simulink model "VTOLTiltrotor"  (R2024b)
settings: configuration reference "VTOLConfiguration" (kept outside this file)
undefined symbols (not defined in the file): airspeed, CityMission, ddx, ddy, ddz, dx, dy, dz, Earth, FixedWingMission, fractalcoef, HoverMission, p, params, pitch, position, q, r, roll, SensorAAFiltDen, SensorAAFiltNum, TransitionMission, UAVSampleTime, WGS84, X, Y, yaw, Z
libraries: robotcorelib x3, simulink x2, mspfiltlib x1, simulink_extras x1, aerolibtransform2 x1, aerolibatmos2 x1, sensorgpslib x1, mspsensorlib x1, sim3dlib x1, uavsim3dlib x1, uavutilslib x1
settings Model: DataDictionary=VTOLDynamicsData.sldd  PauseTimes=13.8  Creator=The MathWorks, Inc.  LastModifiedBy=mhcho
settings ConfigSetRef: SourceName=VTOLConfiguration

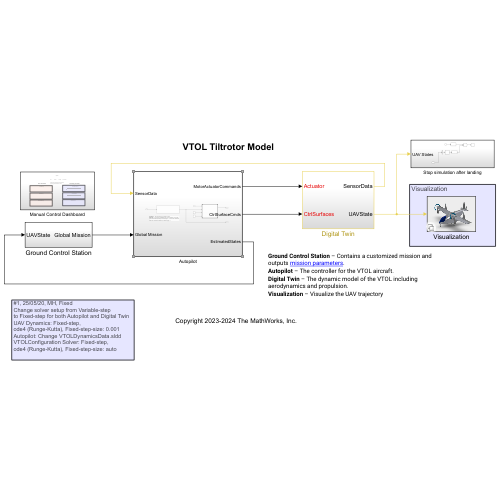
[thumbnail: Simulink's stored preview of the top-level diagram]
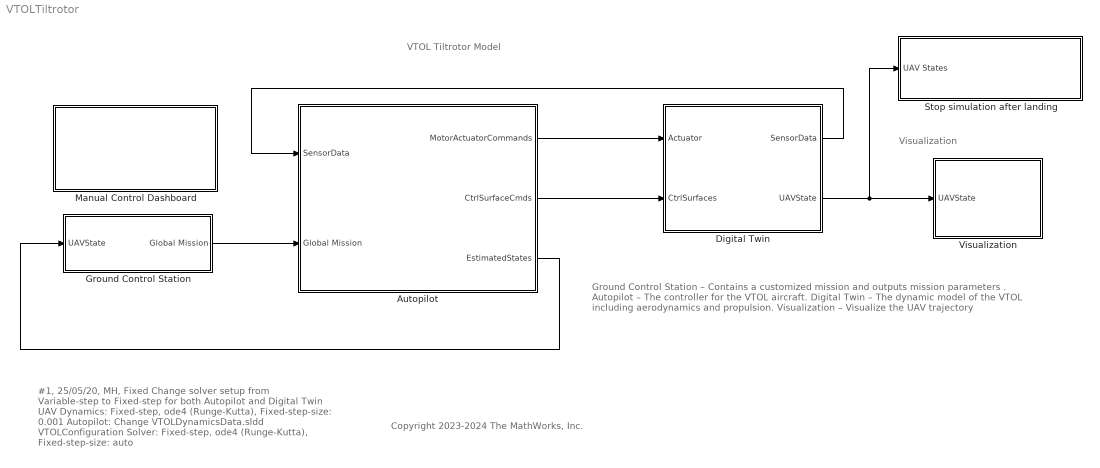
== system VTOLTiltrotor ==
  note: Ground Control Station – Contains a customized mission and outputs mission parameters .
      | Autopilot – The controller for the VTOL aircraft.
      | Digital Twin – The dynamic model of the VTOL including aerodynamics and propulsion.
      | Visualization – Visualize the UAV trajectory
  note: VTOL Tiltrotor Model
  note: Visualization
  note: Copyright 2023-2024 The MathWorks, Inc.
  note: #1, 25/05/20, MH, Fixed
      | Change solver setup from Variable-step
      | to Fixed-step for both Autopilot and Digital Twin
      | UAV Dynamics: Fixed-step,
      | ode4 (Runge-Kutta), Fixed-step-size: 0.001
      | Autopilot: Change VTOLDynamicsData.sldd
      | VTOLConfiguration Solver: Fixed-step,
      | ode4 (Runge-Kutta), Fixed-step-size: auto
  Autopilot : Subsystem
  Digital Twin : Subsystem
  Ground Control Station : Subsystem
  Manual Control Dashboard : Subsystem
  Stop simulation after landing : Subsystem
  Visualization : Subsystem  Variant=on  VariantControl=Visualization
      mask Display: image('TiltrotorVisualization.PNG'); % Use "Edit Image" on toolstrip to change.
  wires:
  Digital Twin/2(UAVState) -> Stop simulation after landing/1(UAV States), Visualization/1(UAVState)
  Ground Control Station/1(Global Mission) -> Autopilot/2(Global Mission)
  Autopilot/3(EstimatedStates) -> Ground Control Station/1(UAVState)
  Digital Twin/1(SensorData) -> Autopilot/1(SensorData)
  Autopilot/1(MotorActuatorCommands) -> Digital Twin/1(Actuator)
  Autopilot/2(CtrlSurfaceCmds) -> Digital Twin/2(CtrlSurfaces)

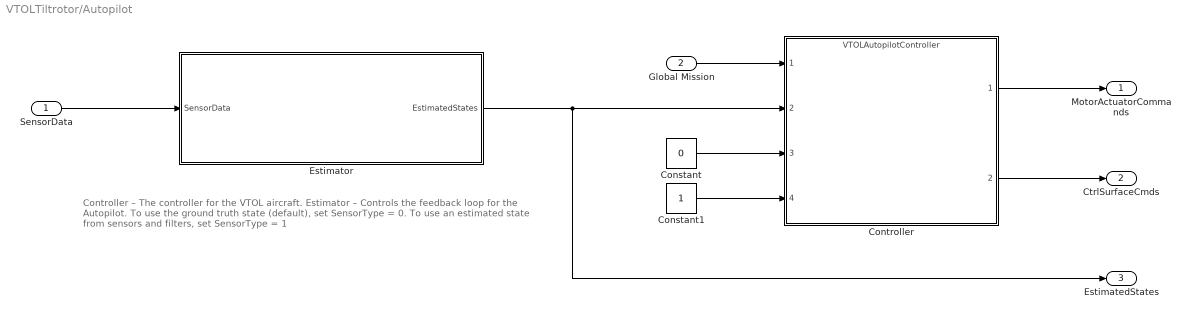
== system VTOLTiltrotor/Autopilot ==
  note: Controller – The controller for the VTOL aircraft.
      | Estimator – Controls the feedback loop for the Autopilot. To use the ground truth state (default), set SensorType = 0. To use an estimated state from sensors and filters, set SensorType = 1
  SensorData : Inport
  Global Mission : Inport  Port=2
  Constant : Constant  Value=0
  Constant1 : Constant
  Controller : ModelReference  ModelNameDialog=VTOLAutopilotController  SimulationMode=Normal  ModelReferenceVersion=1.218
  Estimator : Subsystem  Variant=on
  MotorActuatorCommands : Outport
  CtrlSurfaceCmds : Outport  Port=2
  EstimatedStates : Outport  Port=3
  wires:
  Estimator/1(EstimatedStates) -> EstimatedStates/1, Controller/2
  Controller/1 -> MotorActuatorCommands/1
  SensorData/1 -> Estimator/1(SensorData)
  Controller/2 -> CtrlSurfaceCmds/1
  Global Mission/1 -> Controller/1
  Constant/1 -> Controller/3
  Constant1/1 -> Controller/4

== system VTOLTiltrotor/Digital Twin ==
  Actuator : Inport
  CtrlSurfaces : Inport  Port=2
  Rate Transition : RateTransition
  Rate Transition1 : RateTransition
  To Workspace : ToWorkspace  VariableName=UAV_State  SaveFormat=Timeseries  SampleTime=-1
  UAV Dynamics : ModelReference  ModelNameDialog=VTOLDynamics  SimulationMode=Normal  ModelReferenceVersion=1.74
  Variant Subsystem : Subsystem  Variant=on  VariantControl=Choice
  SensorData : Outport
  UAVState : Outport  Port=2
  wires:
  Variant Subsystem/1(SensorData) -> SensorData/1
  UAV Dynamics/1 -> To Workspace/1, Variant Subsystem/1(UAVStates), UAVState/1  "Ground Truth"
  Actuator/1 -> Rate Transition/1
  CtrlSurfaces/1 -> Rate Transition1/1
  Rate Transition/1 -> UAV Dynamics/1
  Rate Transition1/1 -> UAV Dynamics/2

== system VTOLTiltrotor/Ground Control Station ==
  note: Set mission type. In the project shortcut, choose between:
      | Hover mission by selecting Guidance Mode under Hover
      | Fixed wing mission by selecting Guidance Mode under Fixed wing
      | Transition mission by selecting Set Up Full Transition Mission under Transition
      | City mission by selecting Set Up City Mission under Photorealistic Simulation
  UAVState : Inport
  Get Flight Mission : Subsystem  Variant=on  VariantControlMode=label  LabelModeActiveChoice=useQGC==0
  Global Mission : Outport  SampleTime=0.005
  wires:
  UAVState/1 -> Get Flight Mission/1(UAVState)
  Get Flight Mission/1("Mission ") -> Global Mission/1

== system VTOLTiltrotor/Manual Control Dashboard ==
  note: Commanded Altitude
  note: Flight Mode
  note: Commanded Y (m)
  note: Fixed Wing
  note: Commanded Airspeed (m)
  note: Hover
  note: Transition
  note: Commanded Course
  note: Fixed Wing Commands
  note: Hover Commands
  note: Commanded Altitude (m)
  note: Back Transition
  note: Commanded X (m)
  note: Change these parameters during simulation when using manual testbench mode.
  FlightModeSlider : SliderBlock  LabelPosition=Hide  ScaleMax=3  TickInterval=1
  Slider1 : SliderBlock  LabelPosition=Hide  ScaleMax=50  TickInterval=5
  Slider2 : SliderBlock  LabelPosition=Hide  ScaleMin=-30  ScaleMax=30  TickInterval=5
  Slider3 : SliderBlock  LabelPosition=Hide  ScaleMin=-30  ScaleMax=30  TickInterval=5
  Slider5 : SliderBlock  LabelPosition=Hide  ScaleMin=-30  ScaleMax=30  TickInterval=5
  Slider6 : SliderBlock  LabelPosition=Hide  ScaleMin=-100  TickInterval=10
  Slider7 : SliderBlock  LabelPosition=Hide  ScaleMin=10  ScaleMax=30  TickInterval=5

== system VTOLTiltrotor/Stop simulation after landing ==
  UAV States : Inport
  AND : Logic  IconShape=distinctive  AllPortsSameDT=off  OutDataTypeStr=boolean
  Bus Selector : BusSelector  OutputSignals=Xe
  Clock : Clock
  Compare To Constant : simulink/Logic and Bit Operations/Compare To Constant  relop=>=  const=-1e-2  OutDataTypeStr=boolean
  Compare To Constant1 : simulink/Logic and Bit Operations/Compare To Constant  relop=>=  const=5  OutDataTypeStr=boolean
  Selector : Selector  InputPortWidth=3  IndexOptions=Index vector (dialog)  Indices=3  OutputSizes=1
  Stop Simulation : Stop
  wires:
  Bus Selector/1 -> Selector/1  "<Xe>"
  AND/1 -> Stop Simulation/1
  Compare To Constant1/1 -> AND/1
  UAV States/1 -> Bus Selector/1
  Clock/1 -> Compare To Constant1/1
  Compare To Constant/1 -> AND/2
  Selector/1 -> Compare To Constant/1

== system VTOLTiltrotor/Visualization ==
  UAVState : Inport
  No Visualization : Subsystem  VariantControl=Visualization==0
  Photorealistic : Subsystem  VariantControl=Visualization==2
  Visualization : Subsystem  VariantControl=Visualization==1

== system VTOLTiltrotor/Autopilot/Estimator ==
  SensorData : Inport
  Estimation Filter : Subsystem  VariantControl=SensorType==1
  Ground Truth : Subsystem  VariantControl=SensorType==0
  EstimatedStates : Outport

== system VTOLTiltrotor/Digital Twin/Variant Subsystem ==
  UAVStates : Inport
  No Sensors : Subsystem  VariantControl=SensorType==0
  Sensors : Subsystem  VariantControl=SensorType==1
  SensorData : Outport

== system VTOLTiltrotor/Ground Control Station/Get Flight Mission ==
  UAVState : Inport
  noQGC : Subsystem  TreatAsAtomicUnit=on  SystemSampleTime=UAVSampleTime*4  VariantControl=useQGC==0
  "Mission " : Outport

== system VTOLTiltrotor/Visualization/No Visualization ==
  UAVState : Inport
  Terminator : Terminator
  wires:
  UAVState/1 -> Terminator/1

== system VTOLTiltrotor/Visualization/Photorealistic ==
  UAVState : Inport
  Bus Creator : BusCreator  Inputs=6
  Bus Selector : BusSelector  OutputSignals=Euler,Xe
  Demux : Demux  Outputs=3
  Demux1 : Demux  Outputs=3
  Prepare UAV Data : Subsystem
  Simulation 3D Scene Configuration : sim3dlib/Simulation 3D Scene Configuration  Priority=0  ProjectFormat=Unreal Editor  SceneDesc=US city block  ProjectName=I:\29\vdubey.MergedFixedWingReview\matlab\toolbox\shared\sim3d_projects\automotive_project_windows\UE\WindowsNoEditor\VehicleSimulation.exe  ScenePath=/Game/Maps/USCityBlock  UEProjPath=C:\project\AutoVrtlEnv\AutoVrtlEnv.uproject  EnableOpenDRIVE=off  vehTagList={'Custom';'Scene Origin';'VTOL_Vehicle'}  vehTag=VTOL_Vehicle  FreeCameraInitialTranslation=[0, 0, 0]  FreeCameraDefaultInitialTranslation=[-6, 0, 2]  FreeCameraInitialRotation=[0, 0, 0]  FreeCameraDefaultInitialRotation=[0, -15, 0]  OpVisEn=off  Ts=1/10  EnableWindow=on  EnableRemoteAccess=off  EnableWeather=off  SunAzimuth=90  SunAltitude=40.0  EnableGeospatialSun=off  Latitude=0  Longitude=0  Date=2023-01-01  Time=10:30:00  GeoTimeZone=-5.0  SunDaylightSaving=off  wind=1  clouds=10  EnableVolumetricClouds=off  CloudCoverage=0  CloudAltitude=6  fog=0  rain=0  RaindropsEffect=off  SnowDensity=0  EnableGeospatial=off  UseTrueOrigin=off  OriginHeight=200  OriginLatitude=40.744652  OriginLongitude=-73.988864  MapStyle=Aerial  AdditionalAssetIDs=[]  UseAdvancedSunSky=off  SolarTime=11  TimeZone=-5  Day=21  Month=9  Year=2022  UseDaylightSavingTime=on  DSTStartDay=10  DSTStartMonth=3  DSTEndDay=3  DSTEndMonth=11  DSTSwitchHour=2  sensorTag=MainCamera2  sensorId=2  sensorName=MainCamera2  mountLoc=Origin  offsetFlag=off  tmountOffset=[0, 0, 0]  rmountOffset=[0, 0, 0]  HorizontalResolution=1280  VerticalResolution=720  HorizontalFOV=60  mountPoint=[0 0 0]  mountOrientation=[0 0 0]  aMode=4  ID=2  GeoTrigger=Inactive
      settings: LibrarySourceBlock=uavsim3dlib/Simulation 3D Scene Configuration
  Simulation 3D UAV Vehicle : uavsim3dlib/Simulation 3D UAV Vehicle  Priority=-1  Mesh=Custom  MeshPath=SkeletalMesh'/Game/Maps/VTOLDEMO/VTOLAsset.VTOLAsset'  Color=Black  ActorName=VTOL_Vehicle  UseGlobalFrame=off  InitialTranslation=[0 0 0]  InitialRotation=[0 0 0]  InitialTranslationGlobal=[0 0 0]  InitialGeoOrigin=[0 0 0]  InitialRotationGlobal=[0 0 0]  SampleTime=0.1  ActorType=SimulinkVehicle  ID=C  aMode=4  ActorTag=VTOL_Vehicle
  wires:
  UAVState/1 -> Bus Selector/1
  Bus Selector/2 -> Demux1/1  "<Xe>"
  Bus Selector/1 -> Demux/1  "<Euler>"
  Prepare UAV Data/2(Rotation) -> Simulation 3D UAV Vehicle/2
  Demux/1 -> Bus Creator/1  "roll"
  Demux/3 -> Bus Creator/3  "yaw"
  Demux1/1 -> Bus Creator/4  "x"
  Demux1/2 -> Bus Creator/5  "y"
  Bus Creator/1 -> Prepare UAV Data/1(UAVState)
  Demux1/3 -> Bus Creator/6  "z"
  Demux/2 -> Bus Creator/2  "pitch"
  Prepare UAV Data/1(Translation) -> Simulation 3D UAV Vehicle/1

== system VTOLTiltrotor/Visualization/Visualization ==
  UAVState : Inport
  Bus Selector : BusSelector  OutputSignals=Xe,q,RotorParameters.Tilt1,RotorParameters.Tilt2
  Gain : Gain  Gain=0
  Subsystem : Subsystem
  Trajectory : uavutilslib/UAV Animation  NumUAV=1  DynamicUAVConfig=off  UAVType=FixedWing  UAVSize=5  UAVColor=[1 0 0]  UAVTrajectoryAlpha=1  InertialZDirection=Down  RotationFormat=Quaternion  DrawMarkers=off  SampleTime=0.1
  wires:
  Bus Selector/2 -> Subsystem/2(<q>), Trajectory/2  "<q>"
  Bus Selector/1 -> Trajectory/1, Gain/1  "<Xe>"
  Gain/1 -> Subsystem/1(<Xe>)
  UAVState/1 -> Bus Selector/1
  Bus Selector/3 -> Subsystem/3(RotorA)  "<Tilt1>"
  Bus Selector/4 -> Subsystem/4(RotorB)  "<Tilt2>"

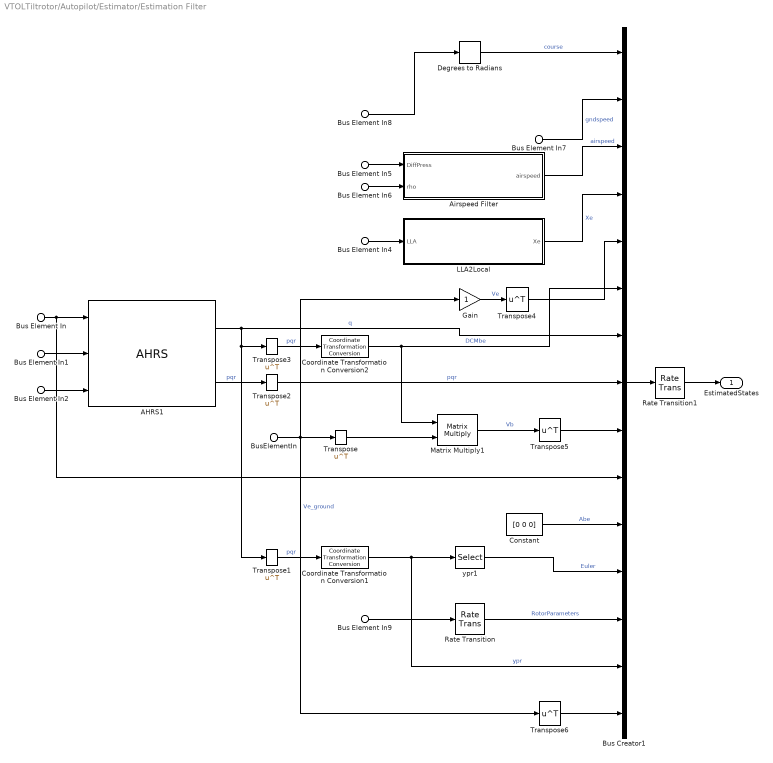
== system VTOLTiltrotor/Autopilot/Estimator/Estimation Filter ==
  Bus Element In : Inport  PortName=SensorData  Element=Abb
  Bus Element In1 : Inport  PortName=SensorData  Element=Gyro
  Bus Element In2 : Inport  PortName=SensorData  Element=Mag
  Bus Element In4 : Inport  PortName=SensorData  Element=LLA
  Bus Element In6 : Inport  PortName=SensorData  Element=rho
  Bus Element In5 : Inport  PortName=SensorData  Element=DiffPress
  Bus Element In7 : Inport  PortName=SensorData  Element=GPSGroundSpeed
  Bus Element In8 : Inport  PortName=SensorData  Element=GPSCourse
  Bus Element In9 : Inport  PortName=SensorData  Element=RotorParameters
  BusElementIn : Inport  PortName=SensorData  Element=GPSVelocity
  AHRS1 : mspfiltlib/AHRS  DispRefFrame=NED  DecimationFactor=1  InitialProcessNoise=ahrsfilter.defaultProcessNoise  OrientationFormat=quaternion  SimulateUsing=Code generation  AccelerometerNoise=0.0001924722  GyroscopeNoise=9.1385e-5  MagnetometerNoise=0.1  GyroscopeDriftNoise=3.0462e-13  LinearAccelerationNoise=0.0096236100000000012  MagneticDisturbanceNoise=0.5  LinearAccelerationDecayFactor=0.998  MagneticDisturbanceDecayFactor=0.5  ExpectedMagneticFieldStrength=40
  Airspeed Filter : Subsystem
  Bus Creator1 : BusCreator  Inputs=15  OutDataTypeStr=Bus: stateBus  NonVirtualBus=on
      settings: InheritFromInputs=off
  Constant : Constant  Value=[0 0 0]
  Coordinate Transformation Conversion1 : robotcorelib/Coordinate Transformation Conversion  InputRepresentation=Quaternion  InputEulerSequence=ZYX  ShowTrVecInputPort=on  OutputRepresentation=Euler Angles  OutputEulerSequence=ZYX  ShowTrVecOutputPort=on  SimulateUsing=Interpreted execution
      settings: LibrarySourceBlock=navlib/Utilities/Coordinate Transformation Conversion
  Coordinate Transformation Conversion2 : robotcorelib/Coordinate Transformation Conversion  InputRepresentation=Quaternion  InputEulerSequence=ZYX  ShowTrVecInputPort=on  OutputRepresentation=Rotation Matrix  OutputEulerSequence=ZYX  ShowTrVecOutputPort=on  SimulateUsing=Interpreted execution
      settings: LibrarySourceBlock=navlib/Utilities/Coordinate Transformation Conversion
  Degrees to Radians : simulink_extras/Transformations/Degrees to Radians
  Gain : Gain
  LLA2Local : Subsystem
  Matrix Multiply1 : Product  Multiplication=Matrix(*)
  Rate Transition : RateTransition  OutPortSampleTime=0.001
  Rate Transition1 : RateTransition
  Transpose{,1..6} (7 alike) : Math  Operator=transpose
  ypr1 : Selector  InputPortWidth=3  IndexOptions=Index vector (dialog)  Indices=[3 2 1]  OutputSizes=1
  EstimatedStates : Outport
  wires:
  Bus Element In1/1 -> AHRS1/2
  Bus Element In/1 -> Bus Creator1/10, AHRS1/1
  Transpose/1 -> Matrix Multiply1/2
  Bus Element In2/1 -> AHRS1/3
  Bus Element In6/1 -> Airspeed Filter/2(rho)
  Transpose2/1 -> Bus Creator1/8  "pqr"
  Transpose3/1 -> Coordinate Transformation Conversion2/1  "pqr"
  AHRS1/1 -> Transpose3/1, Transpose1/1, Bus Creator1/7  "q"
  Airspeed Filter/1(airspeed) -> Bus Creator1/3  "airspeed"
  AHRS1/2 -> Transpose2/1  "pqr"
  BusElementIn/1 -> Transpose6/1, Transpose/1, Gain/1  "Ve_ground"
  Transpose1/1 -> Coordinate Transformation Conversion1/1  "pqr"
  Bus Element In8/1 -> Degrees to Radians/1
  Bus Element In4/1 -> LLA2Local/1(LLA)
  Bus Element In5/1 -> Airspeed Filter/1(DiffPress)
  Coordinate Transformation Conversion2/1 -> Bus Creator1/6, Matrix Multiply1/1  "DCMbe"
  Rate Transition1/1 -> EstimatedStates/1
  Coordinate Transformation Conversion1/1 -> Bus Creator1/14, ypr1/1  "ypr"
  Bus Element In9/1 -> Rate Transition/1
  Degrees to Radians/1 -> Bus Creator1/1  "course"
  Bus Element In7/1 -> Bus Creator1/2  "gndspeed"
  Rate Transition/1 -> Bus Creator1/13  "RotorParameters"
  LLA2Local/1(Xe) -> Bus Creator1/4  "Xe"
  Matrix Multiply1/1 -> Transpose5/1  "Vb"
  Gain/1 -> Transpose4/1  "Ve"
  Constant/1 -> Bus Creator1/11  "Abe"
  ypr1/1 -> Bus Creator1/12  "Euler"
  Bus Creator1/1 -> Rate Transition1/1
  Transpose4/1 -> Bus Creator1/5
  Transpose5/1 -> Bus Creator1/9
  Transpose6/1 -> Bus Creator1/15

== system VTOLTiltrotor/Autopilot/Estimator/Ground Truth ==
  SensorData : Inport
  Rate Transition : RateTransition  OutPortSampleTime=0.005
  EstimatedStates : Outport
  wires:
  SensorData/1 -> Rate Transition/1
  Rate Transition/1 -> EstimatedStates/1

== system VTOLTiltrotor/Digital Twin/Variant Subsystem/No Sensors ==
  UAVStates : Inport
  Rate Transition : RateTransition  OutPortSampleTime=0.005
  SensorData : Outport
  wires:
  Rate Transition/1 -> SensorData/1
  UAVStates/1 -> Rate Transition/1

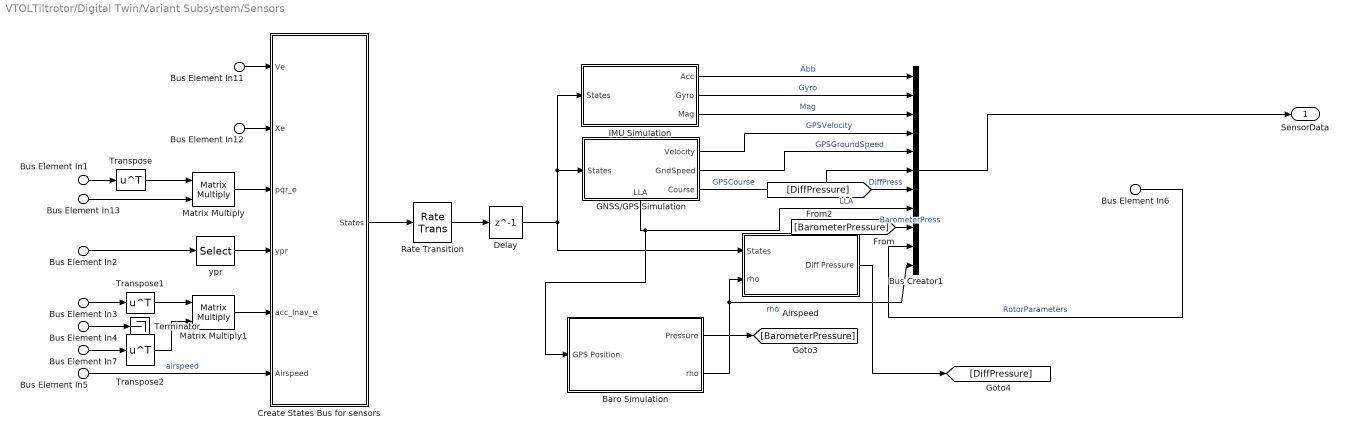
== system VTOLTiltrotor/Digital Twin/Variant Subsystem/Sensors ==
  Bus Element In11 : Inport  PortName=UAVStates  Element=Ve
  Bus Element In12 : Inport  PortName=UAVStates  Element=Xe
  Bus Element In13 : Inport  PortName=UAVStates  Element=pqr
  Bus Element In1 : Inport  PortName=UAVStates  Element=DCMbe
  Bus Element In3 : Inport  PortName=UAVStates  Element=DCMbe
  Bus Element In2 : Inport  PortName=UAVStates  Element=Euler
  Bus Element In4 : Inport  PortName=UAVStates  Element=Abb
  Bus Element In5 : Inport  PortName=UAVStates  Element=airspeed
  Bus Element In6 : Inport  PortName=UAVStates  Element=RotorParameters
  Bus Element In7 : Inport  PortName=UAVStates  Element=Abe
  " Baro Simulation" : Subsystem
  Airspeed : Subsystem
  Bus Creator1 : BusCreator  Inputs=11
  Create States Bus for sensors : Subsystem
  Delay : Delay  DelayLength=1
  GNSS/GPS Simulation : Subsystem
      settings: PortSchema="{\"entries\":[{\"content\":{\"sides\":[{\"content\":{\"connectorIds\":[\"In1\"]},\"type\":\"ConnectorPlacement.EquallySpacedRectSide\",\"uuid\":\"4934e8ff-5d4b-4e11-968d-c23bd62383a0\"},{\"content\":{\"connectorIds\":[\"Out1\",\"Out2\",\"Out3\"],\"side\":\"RIGHT\"},\"type\":\"ConnectorPlacement.EquallySpacedRectSide\",\"uuid\":\"9ec8bc0a-2d3c-4dca-835c-010ac29b6ebc\"},{\"content\":{\"connectorIds\":[],\"side\":\"TOP\"},\"type\":\"ConnectorPlacement.EquallySpacedRectSide\",\"uuid\":\"04f09eb4-1bd9-450e-b951-47054bdd92ad\"},{\"content\":{\"connectorIds\":[\"Out4\"],\"side\":\"BOTTOM\"},\"type\":\"ConnectorPlacement.EquallySpacedRectSide\",\"uuid\":\"54bba437-6d13-4ada-8e8d-b8e04495ee78\"}]},\"type\":\"ConnectorPlacement.EquallySpacedConnector\",\"uuid\":\"9a5920cf-a58d-4c98-839b-fbac94edbe7e\"}],\"packageUris\":[\"http://schema.mathworks.com/mf0/Connector/R2020b\"],\"version\":\"1.0\"}"
  IMU Simulation : Subsystem
  Matrix Multiply : Product  Multiplication=Matrix(*)
  Matrix Multiply1 : Product  Multiplication=Matrix(*)
  Rate Transition : RateTransition  OutPortSampleTime=0.001
  Terminator : Terminator
  Transpose : Math  Operator=transpose
  Transpose1 : Math  Operator=transpose
  Transpose2 : Math  Operator=transpose
  ypr : Selector  InputPortWidth=3  IndexOptions=Index vector (dialog)  Indices=[3 2 1]  OutputSizes=1
  SensorData : Outport
  wires:
  GNSS/GPS Simulation/2(GndSpeed) -> Bus Creator1/5  "GPSGroundSpeed"
  Rate Transition/1 -> Delay/1
  Bus Element In1/1 -> Transpose/1
  Bus Element In13/1 -> Matrix Multiply/2
  IMU Simulation/1(Acc) -> Bus Creator1/1  "Abb"
  IMU Simulation/2(Gyro) -> Bus Creator1/2  "Gyro"
  [BarometerPressure] -> Bus Creator1/9  "BarometerPress"
  Bus Element In11/1 -> Create States Bus for sensors/1(Ve)
  GNSS/GPS Simulation/3(Course) -> Bus Creator1/6  "GPSCourse"
  " Baro Simulation"/2(rho) -> Bus Creator1/11, Airspeed/2(rho)  "rho"
  GNSS/GPS Simulation/4(LLA) -> Bus Creator1/8, " Baro Simulation"/1(GPS Position)  "LLA"
  Transpose1/1 -> Matrix Multiply1/1
  Delay/1 -> IMU Simulation/1(States), GNSS/GPS Simulation/1(States), Airspeed/1(States)
  Bus Element In6/1 -> Bus Creator1/10  "RotorParameters"
  [DiffPressure] -> Bus Creator1/7  "DiffPress"
  Bus Element In12/1 -> Create States Bus for sensors/2(Xe)
  Create States Bus for sensors/1(States) -> Rate Transition/1
  " Baro Simulation"/1(Pressure) -> [BarometerPressure]
  Bus Element In5/1 -> Create States Bus for sensors/6(Airspeed)  "airspeed"
  Matrix Multiply/1 -> Create States Bus for sensors/3(pqr_e)
  GNSS/GPS Simulation/1(Velocity) -> Bus Creator1/4  "GPSVelocity"
  Bus Element In2/1 -> ypr/1
  IMU Simulation/3(Mag) -> Bus Creator1/3  "Mag"
  Bus Element In7/1 -> Transpose2/1
  Airspeed/1(Diff Pressure) -> [DiffPressure]
  Matrix Multiply1/1 -> Create States Bus for sensors/5(acc_lnav_e)
  ypr/1 -> Create States Bus for sensors/4(ypr)
  Bus Element In3/1 -> Transpose1/1
  Transpose/1 -> Matrix Multiply/1
  Bus Element In4/1 -> Terminator/1
  Bus Creator1/1 -> SensorData/1
  Transpose2/1 -> Matrix Multiply1/2

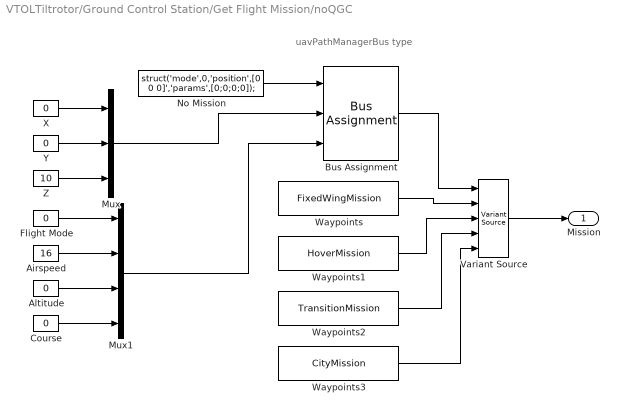
== system VTOLTiltrotor/Ground Control Station/Get Flight Mission/noQGC ==
  note: uavPathManagerBus type
  Airspeed : Constant  Value=16
  Altitude : Constant  Value=0
  Bus Assignment : BusAssignment  AssignedSignals=position,params
  Course : Constant  Value=0
  Flight Mode : Constant  Value=0
  Mux : Mux  Inputs=3
  Mux1 : Mux
  No Mission : Constant  Value=struct('mode',0,'position',[0 0 0]','params',[0;0;0;0]);  OutDataTypeStr=Bus: doubleUavPathManager
  Variant Source : VariantSource
  Waypoints : Constant  Value=FixedWingMission  OutDataTypeStr=Bus: doubleUavPathManager  SampleTime=-1
  Waypoints1 : Constant  Value=HoverMission  OutDataTypeStr=Bus: doubleUavPathManager  SampleTime=-1
  Waypoints2 : Constant  Value=TransitionMission  OutDataTypeStr=Bus: doubleUavPathManager  SampleTime=-1
  Waypoints3 : Constant  Value=CityMission  OutDataTypeStr=Bus: doubleUavPathManager  SampleTime=-1
  X : Constant  Value=0
  Y : Constant  Value=0
  Z : Constant  Value=10
  Mission : Outport
  wires:
  Waypoints/1 -> Variant Source/2
  Waypoints1/1 -> Variant Source/3
  Variant Source/1 -> Mission/1
  Waypoints2/1 -> Variant Source/4
  No Mission/1 -> Bus Assignment/1
  Waypoints3/1 -> Variant Source/5
  Bus Assignment/1 -> Variant Source/1
  X/1 -> Mux/1
  Y/1 -> Mux/2
  Z/1 -> Mux/3
  Mux/1 -> Bus Assignment/2
  Mux1/1 -> Bus Assignment/3
  Flight Mode/1 -> Mux1/1
  Course/1 -> Mux1/4
  Altitude/1 -> Mux1/3
  Airspeed/1 -> Mux1/2

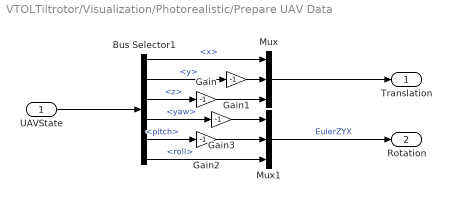
== system VTOLTiltrotor/Visualization/Photorealistic/Prepare UAV Data ==
  UAVState : Inport
  Bus Selector1 : BusSelector  OutputSignals=x,y,z,yaw,pitch,roll
  Gain{,1..3} (4 alike) : Gain  Gain=-1
  Mux : Mux  Inputs=3
  Mux1 : Mux  Inputs=3
  Translation : Outport
  Rotation : Outport  Port=2
  wires:
  UAVState/1 -> Bus Selector1/1
  Mux/1 -> Translation/1
  Mux1/1 -> Rotation/1  "EulerZYX"
  Bus Selector1/4 -> Gain3/1  "<yaw>"
  Bus Selector1/5 -> Gain2/1  "<pitch>"
  Bus Selector1/6 -> Mux1/3  "<roll>"
  Bus Selector1/3 -> Gain/1  "<z>"
  Bus Selector1/2 -> Gain1/1  "<y>"
  Bus Selector1/1 -> Mux/1  "<x>"
  Gain/1 -> Mux/3
  Gain1/1 -> Mux/2
  Gain2/1 -> Mux1/2
  Gain3/1 -> Mux1/1

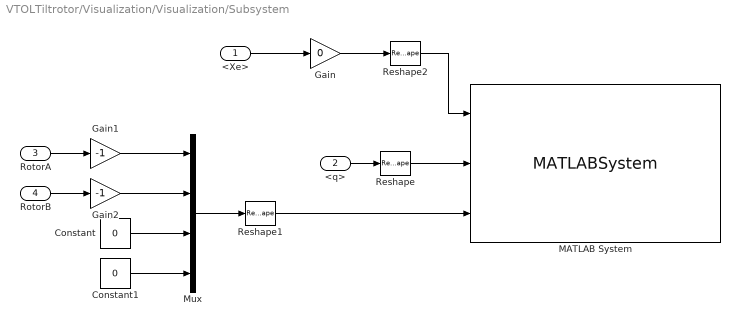
== system VTOLTiltrotor/Visualization/Visualization/Subsystem ==
  <Xe> : Inport
  <q> : Inport  Port=2
  RotorA : Inport  Port=3
  RotorB : Inport  Port=4
  Constant : Constant  Value=0
  Constant1 : Constant  Value=0
  Gain : Gain  Gain=0
  Gain1 : Gain  Gain=-1
  Gain2 : Gain  Gain=-1
  MATLAB System : MATLABSystem  System=exampleHelperTiltRotorAnimator  SampleTime=0.05
      mask Type: exampleHelperTiltRotorAnimator
      mask Display:
      | disp('exampleHelperTiltRotorAnimator');
      | port_label('input',1,'position');
      | port_label('input',2,'orientation');
      | port_label('input',3,'rotorAngles');
  Mux : Mux
  Reshape : Reshape  OutputDimensionality=Customize  OutputDimensions=[1,4]
  Reshape1 : Reshape  OutputDimensionality=Customize  OutputDimensions=[1,4]
  Reshape2 : Reshape  OutputDimensionality=Customize  OutputDimensions=[1,3]
  wires:
  Gain1/1 -> Mux/1
  Constant1/1 -> Mux/4
  Gain2/1 -> Mux/2
  Reshape1/1 -> MATLAB System/3
  Mux/1 -> Reshape1/1
  RotorA/1 -> Gain1/1
  <Xe>/1 -> Gain/1
  Constant/1 -> Mux/3
  RotorB/1 -> Gain2/1
  <q>/1 -> Reshape/1
  Reshape2/1 -> MATLAB System/1
  Reshape/1 -> MATLAB System/2
  Gain/1 -> Reshape2/1

== system VTOLTiltrotor/Autopilot/Estimator/Estimation Filter/Airspeed Filter ==
  DiffPress : Inport
  rho : Inport  Port=2
  Constant : Constant  Value=0.5
  Divide : Product  Inputs=*/
  Product : Product
  Sqrt : Sqrt
  airspeed : Outport
  wires:
  Constant/1 -> Product/2
  rho/1 -> Product/1
  Product/1 -> Divide/2
  DiffPress/1 -> Divide/1
  Divide/1 -> Sqrt/1
  Sqrt/1 -> airspeed/1

== system VTOLTiltrotor/Autopilot/Estimator/Estimation Filter/LLA2Local ==
  LLA : Inport
  Constant1 : Constant  Value=0
  Demux1 : Demux  Outputs=2
  LLA to Flat Earth1 : aerolibtransform2/LLA to Flat Earth  units=Metric (MKS)  ptype=Earth (WGS84)  F=1/298.257223563  R=6378137  refPosPort=off  LL0=[0 0]  psi=0
  Xe : Outport
  wires:
  Constant1/1 -> LLA to Flat Earth1/3
  Demux1/1 -> LLA to Flat Earth1/1
  Demux1/2 -> LLA to Flat Earth1/2
  LLA to Flat Earth1/1 -> Xe/1  "Xe"
  LLA/1 -> Demux1/1

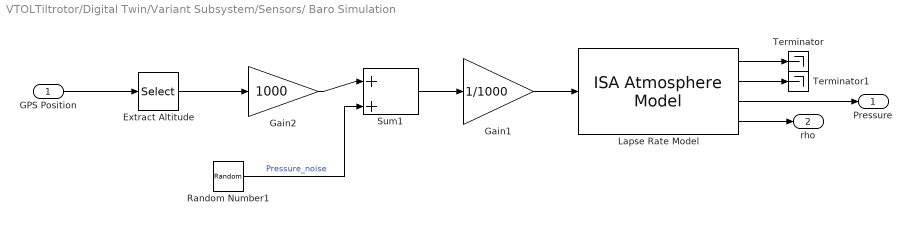
== system VTOLTiltrotor/Digital Twin/Variant Subsystem/Sensors/ Baro Simulation ==
  GPS Position : Inport
  Extract Altitude : Selector  InputPortWidth=3  IndexOptions=Index vector (dialog)  Indices=[3]  OutputSizes=1
  Gain1 : Gain  Gain=1/1000
  Gain2 : Gain  Gain=1000
  Lapse Rate Model : aerolibatmos2/ISA Atmosphere Model  useExtended=off  action=Warning  custom=on  viscosityOut=off  g=9.80665  gamma=1.4  R=287.0531  L=0.0065  h_trop=11000  h_strat=20000  rho0=1.225  P0=101325  T0=288.15  h0=0  S=110.4  Tref=273.15  muref=1.716e-5
  Random Number1 : RandomNumber  Variance=10  Seed=10  SampleTime=.1
  Sum1 : Sum  Inputs=|++
  Terminator : Terminator
  Terminator1 : Terminator
  Pressure : Outport
  rho : Outport  Port=2
  wires:
  Lapse Rate Model/2 -> Terminator1/1
  Lapse Rate Model/4 -> rho/1
  Lapse Rate Model/1 -> Terminator/1
  Lapse Rate Model/3 -> Pressure/1
  Sum1/1 -> Gain1/1
  Gain2/1 -> Sum1/1
  Extract Altitude/1 -> Gain2/1
  Gain1/1 -> Lapse Rate Model/1
  GPS Position/1 -> Extract Altitude/1
  Random Number1/1 -> Sum1/2  "Pressure_noise"

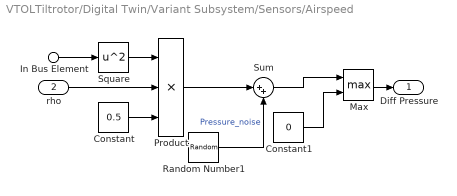
== system VTOLTiltrotor/Digital Twin/Variant Subsystem/Sensors/Airspeed ==
  In Bus Element : Inport  PortName=States  Element=airspeed
  rho : Inport  Port=2
  Constant : Constant  Value=0.5
  Constant1 : Constant  Value=0
  Max : MinMax  Function=max  Inputs=2
  Product : Product  Inputs=3
  Random Number1 : RandomNumber  Variance=0.1  Seed=545  SampleTime=.1
  Square : Math  Operator=square
  Sum : Sum  Inputs=|++
  Diff Pressure : Outport
  wires:
  Constant/1 -> Product/3
  rho/1 -> Product/2
  Square/1 -> Product/1
  In Bus Element/1 -> Square/1
  Product/1 -> Sum/1
  Random Number1/1 -> Sum/2  "Pressure_noise"
  Max/1 -> Diff Pressure/1
  Sum/1 -> Max/1
  Constant1/1 -> Max/2

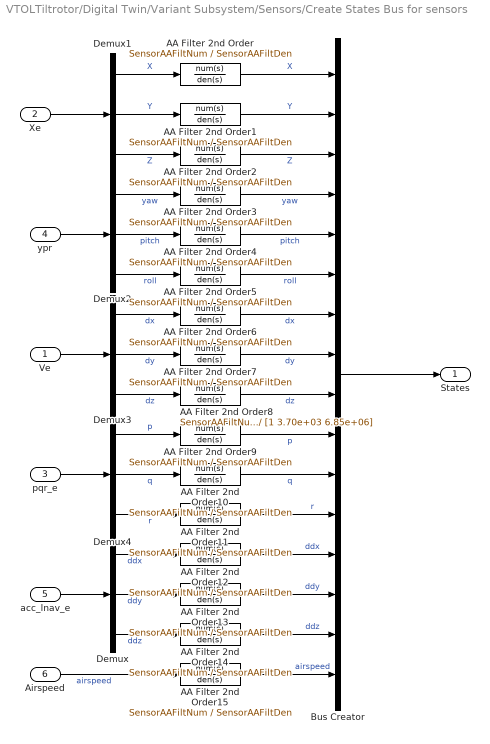
== system VTOLTiltrotor/Digital Twin/Variant Subsystem/Sensors/Create States Bus for sensors ==
  Ve : Inport
  Xe : Inport  Port=2
  pqr_e : Inport  Port=3
  ypr : Inport  Port=4
  acc_lnav_e : Inport  Port=5
  Airspeed : Inport  Port=6
  AA Filter 2nd Order{,1..7,9..15} (15 alike) : TransferFcn  Numerator=SensorAAFiltNum  Denominator=SensorAAFiltDen
  AA Filter 2nd Order8 : TransferFcn  Numerator=SensorAAFiltNum  Denominator=[1 3.70e+03 6.85e+06]
  Bus Creator : BusCreator  Inputs=X,Y,Z,yaw,pitch,roll,dx,dy,dz,p,q,r,ddx,ddy,ddz,airspeed
  Demux{,1..4} (5 alike) : Demux  Outputs=3
  States : Outport
  wires:
  acc_lnav_e/1 -> Demux/1
  pqr_e/1 -> Demux4/1
  Ve/1 -> Demux3/1
  ypr/1 -> Demux2/1
  Xe/1 -> Demux1/1
  Bus Creator/1 -> States/1
  Demux3/3 -> AA Filter 2nd Order8/1  "dz"
  Demux1/3 -> AA Filter 2nd Order2/1  "Z"
  Demux3/2 -> AA Filter 2nd Order7/1  "dy"
  Demux1/2 -> AA Filter 2nd Order1/1  "Y"
  Demux3/1 -> AA Filter 2nd Order6/1  "dx"
  Demux1/1 -> AA Filter 2nd Order/1  "X"
  Demux/1 -> AA Filter 2nd Order12/1  "ddx"
  Demux4/1 -> AA Filter 2nd Order9/1  "p"
  Demux2/1 -> AA Filter 2nd Order3/1  "yaw"
  Demux/2 -> AA Filter 2nd Order13/1  "ddy"
  Demux2/2 -> AA Filter 2nd Order4/1  "pitch"
  Demux/3 -> AA Filter 2nd Order14/1  "ddz"
  Demux2/3 -> AA Filter 2nd Order5/1  "roll"
  Demux4/2 -> AA Filter 2nd Order10/1  "q"
  Demux4/3 -> AA Filter 2nd Order11/1  "r"
  Airspeed/1 -> AA Filter 2nd Order15/1  "airspeed"
  AA Filter 2nd Order/1 -> Bus Creator/1  "X"
  AA Filter 2nd Order1/1 -> Bus Creator/2  "Y"
  AA Filter 2nd Order2/1 -> Bus Creator/3  "Z"
  AA Filter 2nd Order3/1 -> Bus Creator/4  "yaw"
  AA Filter 2nd Order4/1 -> Bus Creator/5  "pitch"
  AA Filter 2nd Order5/1 -> Bus Creator/6  "roll"
  AA Filter 2nd Order6/1 -> Bus Creator/7  "dx"
  AA Filter 2nd Order7/1 -> Bus Creator/8  "dy"
  AA Filter 2nd Order8/1 -> Bus Creator/9  "dz"
  AA Filter 2nd Order9/1 -> Bus Creator/10  "p"
  AA Filter 2nd Order10/1 -> Bus Creator/11  "q"
  AA Filter 2nd Order11/1 -> Bus Creator/12  "r"
  AA Filter 2nd Order12/1 -> Bus Creator/13  "ddx"
  AA Filter 2nd Order13/1 -> Bus Creator/14  "ddy"
  AA Filter 2nd Order14/1 -> Bus Creator/15  "ddz"
  AA Filter 2nd Order15/1 -> Bus Creator/16  "airspeed"

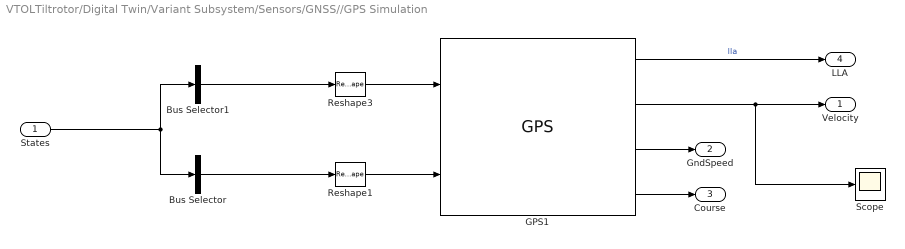
== system VTOLTiltrotor/Digital Twin/Variant Subsystem/Sensors/GNSS//GPS Simulation ==
  States : Inport
  Bus Selector : BusSelector  OutputSignals=dx,dy,dz  OutputAsBus=on
  Bus Selector1 : BusSelector  OutputSignals=X,Y,Z  OutputAsBus=on
  GPS1 : sensorgpslib/GPS  DispRefFrame=NED  PositionInputFormat=Local  ReferenceLocation=[0 0 0]  HorizontalPositionAccuracy=0.01  VerticalPositionAccuracy=0.01  VelocityAccuracy=0.01  DecayFactor=0  SeedDouble=67  SimulateUsing=Code generation
  Reshape1 : Reshape  OutputDimensionality=Row vector (2-D)
  Reshape3 : Reshape  OutputDimensionality=Row vector (2-D)
  Scope : Scope
  Velocity : Outport
  GndSpeed : Outport  Port=2
  Course : Outport  Port=3
  LLA : Outport  Port=4
  wires:
  Reshape3/1 -> GPS1/1
  GPS1/1 -> LLA/1  "lla"
  Bus Selector1/1 -> Reshape3/1
  Bus Selector/1 -> Reshape1/1
  Reshape1/1 -> GPS1/2
  GPS1/2 -> Scope/1, Velocity/1
  States/1 -> Bus Selector/1, Bus Selector1/1
  GPS1/3 -> GndSpeed/1
  GPS1/4 -> Course/1

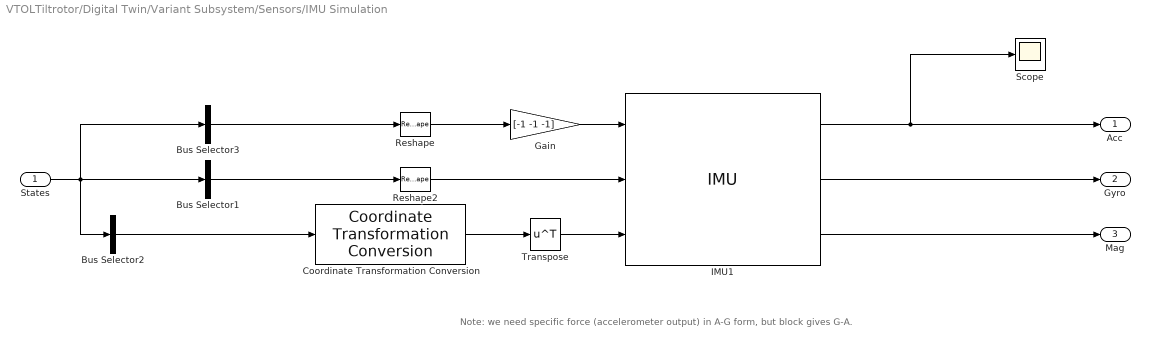
== system VTOLTiltrotor/Digital Twin/Variant Subsystem/Sensors/IMU Simulation ==
  note: Note:
      | we need specific force (accelerometer output) in A-G form, but block gives G-A.
  States : Inport
  Bus Selector1 : BusSelector  OutputSignals=p,q,r  OutputAsBus=on
  Bus Selector2 : BusSelector  OutputSignals=yaw,pitch,roll  OutputAsBus=on
  Bus Selector3 : BusSelector  OutputSignals=ddx,ddy,ddz  OutputAsBus=on
  Coordinate Transformation Conversion : robotcorelib/Coordinate Transformation Conversion  InputRepresentation=Euler Angles  InputEulerSequence=ZYX  ShowTrVecInputPort=on  OutputRepresentation=Rotation Matrix  OutputEulerSequence=ZYX  ShowTrVecOutputPort=on  SimulateUsing=Code generation
  Gain : Gain  Gain=[-1 -1 -1]
  IMU1 : mspsensorlib/IMU  DispRefFrame=NED  TemperaturePort=off  Temperature=25  MagneticFieldPort=off  MagneticFieldNED=[27.5550,-2.4169,-16.0849]  MagneticFieldENU=[ -2.4169, 27.5550, 16.0849 ]  SeedDouble=87254  SimulateUsing=Code generation  AccelParamsMeasurementRange=Inf  AccelParamsResolution=0  AccelParamsConstantBias=[ 0, 0, 0 ]  AccelParamsAxesMisalignment=[ 0, 0, 0 ]  AccelParamsNoiseDensity=0.0003  AccelParamsBiasInstability=[ 0, 0, 0 ]  AccelParamsBiasInstabilityNumerator=fractalcoef().Numerator  AccelParamsBiasInstabilityDenominator=fractalcoef().Denominator  AccelParamsRandomWalk=[ 0, 0, 0 ]  AccelParamsNoiseType=double-sided  AccelParamsTemperatureBias=[ 0, 0, 0 ]  AccelParamsTemperatureScaleFactor=[ 0, 0, 0 ]  GyroParamsMeasurementRange=Inf  GyroParamsResolution=0  GyroParamsConstantBias=[ 0, 0, 0 ]  GyroParamsAxesMisalignment=[ 0, 0, 0 ]  GyroParamsAccelerationBias=0.0001  GyroParamsNoiseDensity=0.0002  GyroParamsBiasInstability=[ 0, 0, 0 ]  GyroParamsBiasInstabilityNumerator=fractalcoef().Numerator  GyroParamsBiasInstabilityDenominator=fractalcoef().Denominator  GyroParamsRandomWalk=[ 0, 0, 0 ]  GyroParamsNoiseType=double-sided  GyroParamsTemperatureBias=[ 0, 0, 0 ]  GyroParamsTemperatureScaleFactor=[ 0, 0, 0 ]  MagParamsMeasurementRange=Inf  MagParamsResolution=0  MagParamsConstantBias=[ 0, 0, 0 ]  MagParamsAxesMisalignment=[ 0, 0, 0 ]  MagParamsNoiseDensity=0.0005  MagParamsBiasInstability=[ 0, 0, 0 ]  MagParamsBiasInstabilityNumerator=fractalcoef().Numerator  MagParamsBiasInstabilityDenominator=fractalcoef().Denominator  MagParamsRandomWalk=[ 0, 0, 0 ]  MagParamsNoiseType=double-sided  MagParamsTemperatureBias=[ 0, 0, 0 ]  MagParamsTemperatureScaleFactor=[ 0, 0, 0 ]
  Reshape : Reshape  OutputDimensionality=Row vector (2-D)
  Reshape2 : Reshape  OutputDimensionality=Row vector (2-D)
  Scope : Scope
  Transpose : Math  Operator=transpose
  Acc : Outport
  Gyro : Outport  Port=2
  Mag : Outport  Port=3
  wires:
  Reshape/1 -> Gain/1
  Bus Selector3/1 -> Reshape/1
  Bus Selector1/1 -> Reshape2/1
  Bus Selector2/1 -> Coordinate Transformation Conversion/1
  Reshape2/1 -> IMU1/2
  States/1 -> Bus Selector1/1, Bus Selector2/1, Bus Selector3/1
  Coordinate Transformation Conversion/1 -> Transpose/1
  IMU1/1 -> Scope/1, Acc/1
  IMU1/3 -> Mag/1
  IMU1/2 -> Gyro/1
  Gain/1 -> IMU1/1
  Transpose/1 -> IMU1/3
